simulink model "untitled"  (R2023b)
settings: Solver=FixedStepAuto  StartTime=0.0  StopTime=10.0  RelTol=1e-3  EnableMultiTasking=on
libraries: arduinolib x6, simulink x2
settings Model: ExtModeTrigDuration=2  Creator=mehme  LastModifiedBy=mehme
settings OptimizationCC: EnhancedBackFolding=on  PassReuseOutputArgsAs=Individual arguments  ZeroExternalMemoryAtStartup=off  ZeroInternalMemoryAtStartup=off  MaxStackSize=64  OptimizeBlockOrder=speed  DifferentSizesBufferReuse=on  OptimizationCustomize=off  EfficientTunableParamExpr=on
settings DebuggingCC: ParameterTunabilityLossMsg=error
settings HardwareCC: ProdBitPerInt=16  ProdBitPerPointer=16  ProdBitPerSizeT=16  ProdBitPerPtrDiffT=16  ProdLargestAtomicFloat=None  ProdWordSize=8  ProdHWDeviceType=Atmel->AVR
settings SFSimCC: MATLABDynamicMemAlloc=off
settings RTWCC: Description=Embedded Coder  SystemTargetFile=ert.tlc  HardwareBoard=Arduino Uno  TemplateMakefile=ert_default_tmf  Toolchain=Arduino AVR  BuildConfiguration=Faster Runs
settings CodeAppCC: ForceParamTrailComments=on  IgnoreCustomStorageClasses=off  OperatorAnnotations=on  SimulinkDataObjDesc=on  SFDataObjDesc=on  InsertBlockDesc=on
settings ERTTargetCC: SupportContinuousTime=on  SupportVariableSizeSignals=on  ExtModeTransport=3  ExtModeStaticAlloc=on  ExtModeAutomaticAllocSize=off  ExtModeStaticAllocSize=250  ExtModeMexFile=ext_xcp  ExtModeIntrfLevel=Level2 - Open

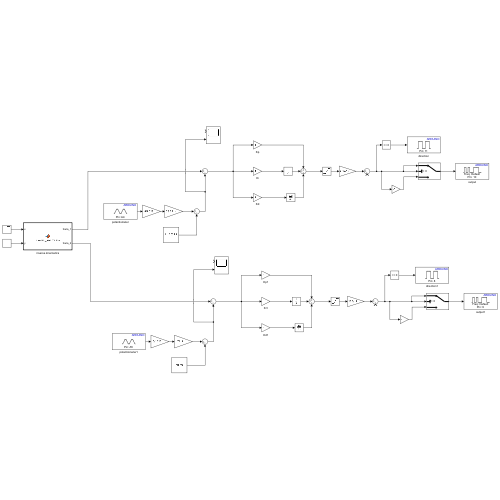
[thumbnail: Simulink's stored preview of the top-level diagram]
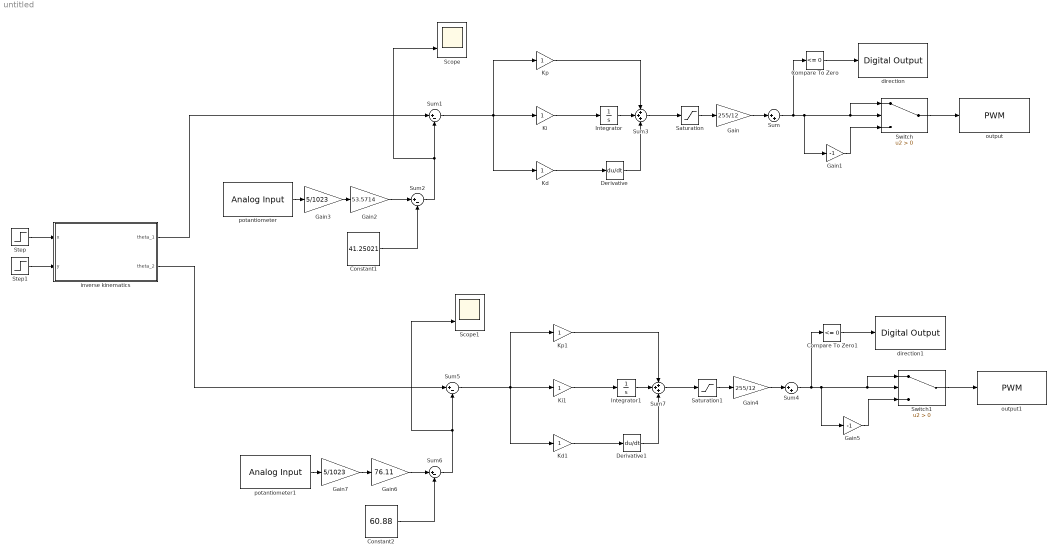
== system untitled ==
  Compare To Zero : simulink/Logic and Bit Operations/Compare To Zero  relop=<=  OutDataTypeStr=boolean
  Compare To Zero1 : simulink/Logic and Bit Operations/Compare To Zero  relop=<=  OutDataTypeStr=boolean
  Constant1 : Constant  Value=41.25021
  Constant2 : Constant  Value=60.88
  Derivative : Derivative
  Derivative1 : Derivative
  Gain : Gain  Gain=255/12
  Gain1 : Gain  Gain=-1
  Gain2 : Gain  Gain=53.5714
  Gain3 : Gain  Gain=5/1023
  Gain4 : Gain  Gain=255/12
  Gain5 : Gain  Gain=-1
  Gain6 : Gain  Gain=76.11
  Gain7 : Gain  Gain=5/1023
  Integrator : Integrator
  Integrator1 : Integrator
  Kd : Gain
  Kd1 : Gain
  Ki : Gain
  Ki1 : Gain
  Kp : Gain
  Kp1 : Gain
  Saturation : Saturate  UpperLimit=12  LowerLimit=-12
  Saturation1 : Saturate  UpperLimit=12  LowerLimit=-12
  Scope : Scope  NumInputPorts=2
  Scope1 : Scope  NumInputPorts=2
  Step : Step  Time=0  After=10  SampleTime=0
  Step1 : Step  Time=0  After=10  SampleTime=0
  Sum : Sum  Inputs=|++
  Sum{1..2,5..6} (4 alike) : Sum  Inputs=|+-
  Sum3 : Sum  Inputs=+++
  Sum4 : Sum  Inputs=|++
  Sum7 : Sum  Inputs=+++
  Switch : Switch  Criteria=u2 > Threshold  SaturateOnIntegerOverflow=off  InputSameDT=off
  Switch1 : Switch  Criteria=u2 > Threshold  SaturateOnIntegerOverflow=off  InputSameDT=off
  direction : arduinolib/Digital Output  pinNumber=11  Direction=output  blockPlatform=arduino
  direction1 : arduinolib/Digital Output  pinNumber=8  Direction=output  blockPlatform=arduino
  inverse kinematics : MATLAB Function  TreatAsAtomicUnit=on
  output : arduinolib/PWM  pinNumber=10  frequencyType=Default  desiredFrequency=490.2  achievableFrequency=490.2
  output1 : arduinolib/PWM  pinNumber=9  frequencyType=Default  desiredFrequency=490.2  achievableFrequency=490.2
  potantiometer : arduinolib/Analog Input  pinNumber=4  ReadResultsOnly=off  ConversionTriggerSource=Software  ExternalTriggerType=uint32( 0 )  OutputDataType=uint16  EnableConversionCompleteNotify=off  EnableOuputStatus=off  SampleTime=-1  blockPlatform=arduino
  potantiometer1 : arduinolib/Analog Input  pinNumber=5  ReadResultsOnly=off  ConversionTriggerSource=Software  ExternalTriggerType=uint32( 0 )  OutputDataType=uint16  EnableConversionCompleteNotify=off  EnableOuputStatus=off  SampleTime=-1  blockPlatform=arduino
  wires:
  Sum3/1 -> Saturation/1
  Integrator/1 -> Sum3/2
  Sum2/1 -> Scope/2, Sum1/2
  Kp/1 -> Sum3/1
  Sum1/1 -> Kd/1, Kp/1, Ki/1
  Derivative/1 -> Sum3/3
  Ki/1 -> Integrator/1
  Sum/1 -> Compare To Zero/1, Gain1/1, Switch/2, Switch/1
  Gain3/1 -> Gain2/1
  Gain1/1 -> Switch/3
  potantiometer/1 -> Gain3/1
  Saturation/1 -> Gain/1
  Kd/1 -> Derivative/1
  Gain2/1 -> Sum2/1
  Gain/1 -> Sum/1
  Compare To Zero/1 -> direction/1
  Constant1/1 -> Sum2/2
  Switch/1 -> output/1
  inverse kinematics/1(theta_1) -> Sum1/1
  Kp1/1 -> Sum7/1
  Sum7/1 -> Saturation1/1
  Gain7/1 -> Gain6/1
  Gain5/1 -> Switch1/3
  Constant2/1 -> Sum6/2
  potantiometer1/1 -> Gain7/1
  Gain6/1 -> Sum6/1
  Kd1/1 -> Derivative1/1
  Switch1/1 -> output1/1
  Compare To Zero1/1 -> direction1/1
  Saturation1/1 -> Gain4/1
  Sum4/1 -> Compare To Zero1/1, Gain5/1, Switch1/2, Switch1/1
  Sum6/1 -> Scope1/2, Sum5/2
  Gain4/1 -> Sum4/1
  Derivative1/1 -> Sum7/3
  Integrator1/1 -> Sum7/2
  Ki1/1 -> Integrator1/1
  Sum5/1 -> Kd1/1, Kp1/1, Ki1/1
  inverse kinematics/2(theta_2) -> Sum5/1
  Step/1 -> inverse kinematics/1(x)
  Step1/1 -> inverse kinematics/2(y)

== matlab function untitled/inverse kinematics ==
  data: x input; theta_1 output; y input; theta_2 output
function [theta_1 , theta_2] = inverse_kinematics(x , y)
a_1 = 2;
a_2 = 5;

theta_2 = -acos((x^2+y^2-a1^2-a2^2)/(2*a1*a2));
theta_1 = atan(y/x) - atan((a2*sin(theta2))/(a1+a2cos(theta2)));
